simulink model "Testing_Modelling_Proportional_Control_In_Laplace_Domain"  (R2020a)
settings: Solver=FixedStepAuto  StartTime=0.0  StopTime=10  FixedStep=0.0001  RelTol=1e-3
values from neighbouring files (symbols this model uses):
  J = 0.005    [motor_parameters.mat]
  Ke = 2.3    [motor_parameters.mat]
  Kf = 0.3    [motor_parameters.mat]
  Kt = 2.19    [motor_parameters.mat]
  L = 1    [motor_parameters.mat]
  R = 1.1    [motor_parameters.mat]
undefined symbols (not defined in the file or in its folder): Kp
settings Model: Creator=alexr  LastModifiedBy=alexr

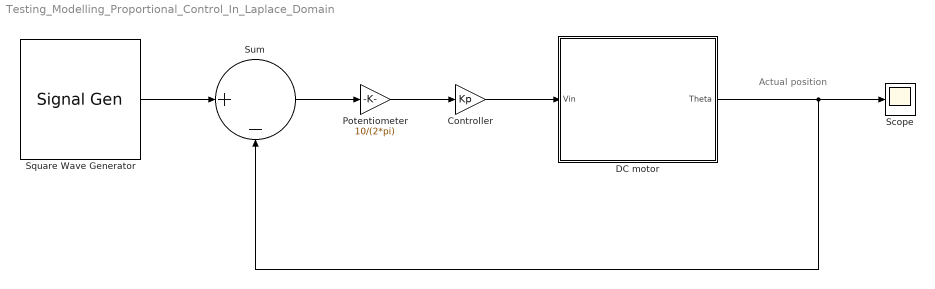
== system Testing_Modelling_Proportional_Control_In_Laplace_Domain ==
  note: Actual position
  Controller : Gain  Gain=Kp
  DC motor : Subsystem
  Potentiometer : Gain  Gain=10/(2*pi)
  Scope : Scope
  Square Wave Generator : SignalGenerator  WaveForm=square  Amplitude=-pi/3  Frequency=pi  Units=rad/sec
  Sum : Sum  Inputs=|+-
  wires:
  Square Wave Generator/1 -> Sum/1
  Controller/1 -> DC motor/1(Vin)
  DC motor/1(Theta) -> Sum/2, Scope/1
  Sum/1 -> Potentiometer/1
  Potentiometer/1 -> Controller/1

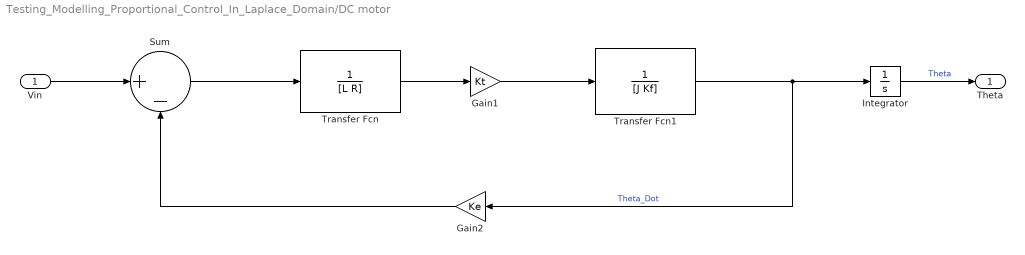
== system Testing_Modelling_Proportional_Control_In_Laplace_Domain/DC motor ==
  Vin : Inport
  Gain1 : Gain  Gain=Kt
  Gain2 : Gain  Gain=Ke
  Integrator : Integrator
  Sum : Sum  Inputs=|+-
  Transfer Fcn : TransferFcn  Denominator=[L R]
  Transfer Fcn1 : TransferFcn  Denominator=[J Kf]
  Theta : Outport
  wires:
  Gain2/1 -> Sum/2
  Transfer Fcn1/1 -> Gain2/1, Integrator/1  "Theta_Dot"
  Sum/1 -> Transfer Fcn/1
  Transfer Fcn/1 -> Gain1/1
  Gain1/1 -> Transfer Fcn1/1
  Vin/1 -> Sum/1
  Integrator/1 -> Theta/1  "Theta"
